simulink model "test_last_update"  (R2018b)
settings: Solver=VariableStepAuto  StartTime=0.0  StopTime=20  RelTol=1e-3
values from neighbouring files (symbols this model uses):
  plane = AirPlane("NT-33A_4.xlsx")    [entryPoint.m]    (also in main.m)
  servo = tf(10,[1 10])    [main.m]
libraries: simulink_extras x4, cstblocks x2
settings Model: Creator=Mo.Hatem  LastModifiedBy=OWNER

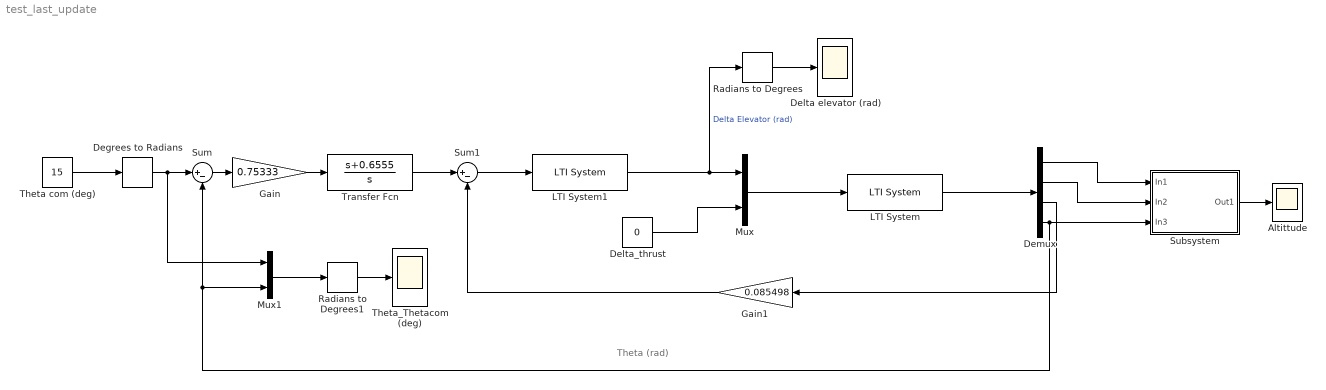
== system test_last_update ==
  note: Theta (rad)
  Altittude : Scope
  Degrees to Radians : simulink_extras/Transformations/Degrees to Radians
  Delta elevator (rad) : Scope
  Delta_thrust : Constant  Value=0
  Demux : Demux
  Gain : Gain  Gain=0.75333
  Gain1 : Gain  Gain=0.085498
  LTI System : cstblocks/LTI System  sys=LongSS  IC=[]
  LTI System1 : cstblocks/LTI System  sys=-servo  IC=[]
  Mux : Mux  Inputs=2
  Mux1 : Mux  Inputs=2
  Radians to Degrees : simulink_extras/Transformations/Radians to Degrees
  Radians to Degrees1 : simulink_extras/Transformations/Radians to Degrees
  Subsystem : Subsystem
  Sum : Sum  Inputs=|+-
  Sum1 : Sum  Inputs=|+-
  Theta com (deg) : Constant  Value=15
  Theta_Thetacom (deg) : Scope
  Transfer Fcn : TransferFcn  Numerator=[1 +0.6555]  Denominator=[1 0]
  wires:
  Mux/1 -> LTI System/1
  LTI System/1 -> Demux/1
  LTI System1/1 -> Radians to Degrees/1, Mux/1  "Delta Elevator (rad)"
  Theta com (deg)/1 -> Degrees to Radians/1
  Degrees to Radians/1 -> Mux1/1, Sum/1
  Demux/4 -> Sum/2, Mux1/2, Subsystem/3(In3)
  Sum/1 -> Gain/1
  Gain/1 -> Transfer Fcn/1
  Transfer Fcn/1 -> Sum1/1
  Sum1/1 -> LTI System1/1
  Demux/3 -> Gain1/1
  Gain1/1 -> Sum1/2
  Delta_thrust/1 -> Mux/2
  Mux1/1 -> Radians to Degrees1/1
  Radians to Degrees/1 -> Delta elevator (rad)/1
  Radians to Degrees1/1 -> Theta_Thetacom (deg)/1
  Demux/1 -> Subsystem/1(In1)
  Demux/2 -> Subsystem/2(In2)
  Subsystem/1(Out1) -> Altittude/1

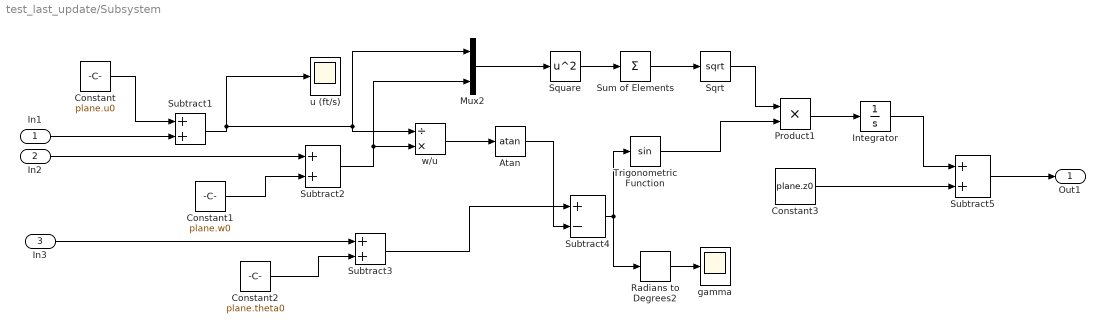
== system test_last_update/Subsystem ==
  In1 : Inport
  In2 : Inport  Port=2
  In3 : Inport  Port=3
  Atan : Trigonometry  Operator=atan
  Constant : Constant  Value=plane.u0
  Constant1 : Constant  Value=plane.w0
  Constant2 : Constant  Value=plane.theta0  VectorParams1D=off
  Constant3 : Constant  Value=plane.z0
  Integrator : Integrator
  Mux2 : Mux  Inputs=2
  Product1 : Product
  Radians to Degrees2 : simulink_extras/Transformations/Radians to Degrees
  Sqrt : Sqrt  SaturateOnIntegerOverflow=on
  Square : Math  Operator=square  SaturateOnIntegerOverflow=on
  Subtract{1..3,5} (4 alike) : Sum
  Subtract4 : Sum  Inputs=+-
  Sum of Elements : Sum  Inputs=+
  Trigonometric Function : Trigonometry
  gamma : Scope
  u (ft/s) : Scope
  w/u : Product  Inputs=/*
  Out1 : Outport
  wires:
  Subtract1/1 -> u (ft/s)/1, w/u/1, Mux2/1
  Mux2/1 -> Square/1
  Atan/1 -> Subtract4/2
  Square/1 -> Sum of Elements/1
  Constant/1 -> Subtract1/1
  Product1/1 -> Integrator/1
  In3/1 -> Subtract3/1
  Constant1/1 -> Subtract2/2
  Subtract2/1 -> w/u/2, Mux2/2
  Sqrt/1 -> Product1/1
  In1/1 -> Subtract1/2
  Subtract5/1 -> Out1/1
  Subtract4/1 -> Trigonometric Function/1, Radians to Degrees2/1
  Constant2/1 -> Subtract3/2
  Sum of Elements/1 -> Sqrt/1
  In2/1 -> Subtract2/1
  Radians to Degrees2/1 -> gamma/1
  Integrator/1 -> Subtract5/1
  Trigonometric Function/1 -> Product1/2
  Subtract3/1 -> Subtract4/1
  Constant3/1 -> Subtract5/2
  w/u/1 -> Atan/1
